simulink model "trc_controller_inout"  (R2019b)
settings: Solver=VariableStepAuto  StartTime=0.0  StopTime=30  RelTol=1e-3
values from neighbouring files (symbols this model uses):
  fl = 1/g    (= 0.0312178066369)    [TRC_Model.m]
  Ki = 0.0095    [TRC_Model.m]
  Kp = 1.351    [TRC_Model.m]
undefined symbols (not defined in the file or in its folder): cf_den, cf_num, DEN, NUM
libraries: simulink_extras x1
settings Model: Creator=Merc  LastModifiedBy=brian
settings SolverCC: ZeroCrossAlgorithm=Adaptive
settings DataIOCC: ReturnWorkspaceOutputs=off
settings DebuggingCC: IgnoredZcDiagnostic=none  ArithmeticOperatorsInVariantConditions=warning
settings SFSimCC: CustomCodeUndefinedFunction=UseInterfaceOnly

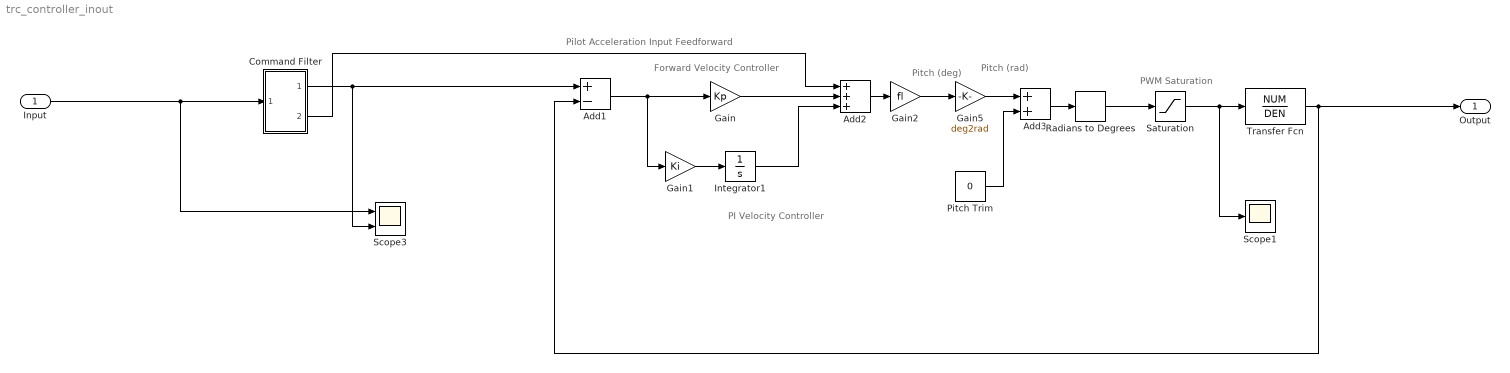
== system trc_controller_inout ==
  note: PWM Saturation
  note: Pitch (rad)
  note: Pitch (deg)
  note: Forward Velocity Controller
  note: PI Velocity Controller
  note: Pilot Acceleration Input Feedforward
  Input : Inport
  Add1 : Sum  Inputs=+-
  Add2 : Sum  Inputs=+++
  Add3 : Sum
  Command Filter : Subsystem
  Gain : Gain  Gain=Kp
  Gain1 : Gain  Gain=Ki
  Gain2 : Gain  Gain=fl
  Gain5 : Gain  Gain=deg2rad
  Integrator1 : Integrator
  Pitch Trim : Constant  Value=0
  Radians to Degrees : simulink_extras/Transformations/Radians to Degrees
  Saturation : Saturate  UpperLimit=400  LowerLimit=-400
  Scope1 : Scope
  Scope3 : Scope  NumInputPorts=2
  Transfer Fcn : TransferFcn  Numerator=NUM  Denominator=DEN
  Output : Outport
  wires:
  Add1/1 -> Gain1/1, Gain/1
  Gain/1 -> Add2/2
  Add2/1 -> Gain2/1
  Pitch Trim/1 -> Add3/2
  Transfer Fcn/1 -> Output/1, Add1/2
  Gain5/1 -> Add3/1
  Gain2/1 -> Gain5/1
  Command Filter/1(Out1) -> Add1/1, Scope3/2
  Command Filter/2(Out2) -> Add2/1
  Add3/1 -> Radians to Degrees/1
  Input/1 -> Scope3/1, Command Filter/1(In1)
  Gain1/1 -> Integrator1/1
  Integrator1/1 -> Add2/3
  Radians to Degrees/1 -> Saturation/1
  Saturation/1 -> Scope1/1, Transfer Fcn/1

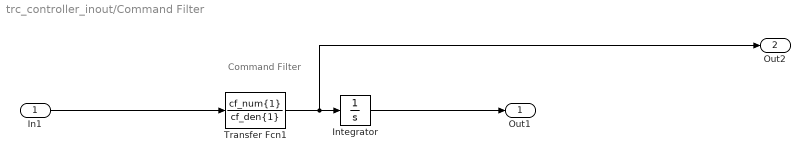
== system trc_controller_inout/Command Filter ==
  note: Command Filter
  In1 : Inport
  Integrator : Integrator
  Transfer Fcn1 : TransferFcn  Numerator=cf_num{1}  Denominator=cf_den{1}
  Out1 : Outport  VectorParamsAs1DForOutWhenUnconnected=off
  Out2 : Outport  Port=2  VectorParamsAs1DForOutWhenUnconnected=off
  wires:
  Integrator/1 -> Out1/1
  In1/1 -> Transfer Fcn1/1
  Transfer Fcn1/1 -> Out2/1, Integrator/1
